simulink model "path_following_PID_v2"  (R2022a)
settings: Solver=VariableStepAuto  StartTime=0.0  StopTime=4000  RelTol=1e-3
model workspace (MAT data in the model file):
  index = 1
values from neighbouring files (symbols this model uses):
  ref = [x_ref, -y_ref]    [reference.m]
libraries: slpidlib x2
settings Model: Creator=andreagottardini  LastModifiedBy=andreagottardini
settings DataIOCC: ReturnWorkspaceOutputs=off

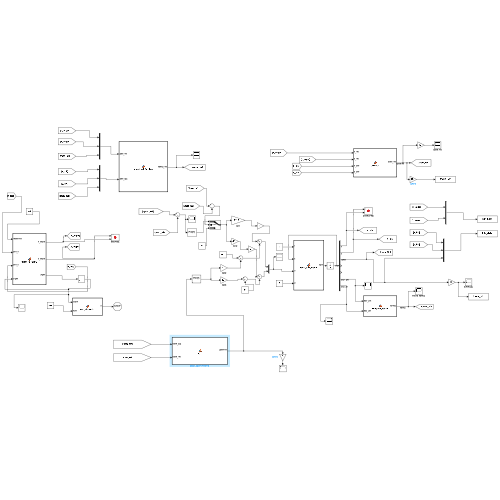
[thumbnail: Simulink's stored preview of the top-level diagram]
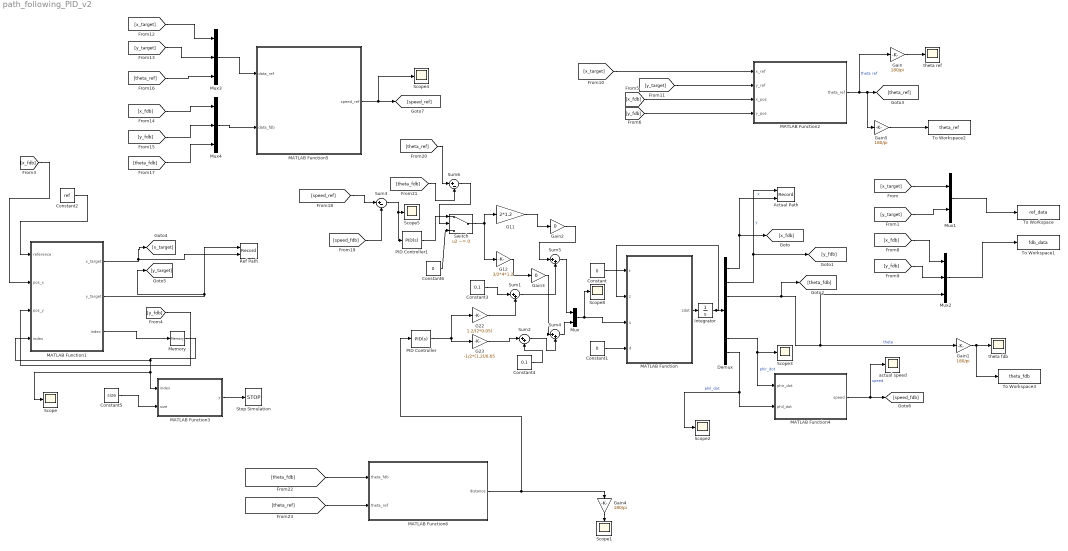
== system path_following_PID_v2 ==
  Actual Path : Record  FileSettingsInternal="{\"entries\":[{\"content\":{\"excelSettings\":{\"content\":{},\"type\":\"Streamout.ExcelSettings\"}},\"type\":\"Streamout.FileSettingStorage\",\"uuid\":\"b8018b94-6d69-4510-834d-5395391f9d9a\"}],\"packageUris\":[\"http://schema.mathworks.com/mf0/streamout_blocks/R2020a\"],\"version\":\"1.0\"}"  Layout=[1 1]  SignalsInternal="{\"entries\":[{\"content\":{\"signals\":[{\"content\":{\"blockPath\":[\"path_following_PID_v2/Actual Path\"],\"channel\":[],\"dimensions\":[1],\"domain\":\"path_following_PID_v2/Actual Path\",\"lineColor\":\"#22b573\",\"plots\":[],\"port\":1,\"sid\":[\"\"],\"signalID\":39276,\"signalName\":\"y\"},\"type\":\"RecordBlkView.Signal\",\"uuid\":\"de93c3ac-fa92-48e5-8615-195f95aa2750\"},{\"content\":{\"blockPath\":[\"path_following_PID_v2/Actual Path\"],\"channel\":[],\"dimensions\":[1],\"domain\":\"path_following_PID_v2/Actual Path\",\"lineColor\":\"#0072bd\",\"plots\":[],\"port\":2,\"sid\":[\"\"],\"signalID\":39280,\"signalName\":\"x\"},\"type\":\"RecordBlkView.Signal\",\"uuid\":\"afc86004-265b-4bb5-8c2d-c825a62d9dd9\"}]},\"type\":\"RecordBlkView.InputSignals\",\"uuid\":\"867639a0-b77e-437d-b3b9-b5e698d5be3f\"}],\"packageUris\":[\"http://schema.mathworks.com/mf0/streamout_blocks/R2020a\"],\"version\":\"1.0\"}"  VisualizationBindings="{\"xyplotplugin\":{\"info\":[{\"series\":[],\"subplotID\":1}]}}"  CompatibilityTag=XY
  Constant : Constant  Value=0
  Constant1 : Constant  Value=0
  Constant2 : Constant  Value=ref
  Constant3 : Constant  Value=0.1
  Constant4 : Constant  Value=0.1
  Constant5 : Constant  Value=size
  Constant6 : Constant  Value=0
  Demux : Demux  Outputs=7
  G11 : Gain  Gain=2*1.2
  G12 : Gain  Gain=3/2*4*1.2
  G22 : Gain  Gain=1.2/(2*0.05)
  G23 : Gain  Gain=-1/2*(1.2)/0.05
  Gain{,1,4..5} (4 alike) : Gain  Gain=180/pi
  Gain2 : Gain  Gain=0
  Gain3 : Gain  Gain=0
  Integrator : Integrator  InitialCondition=[0;0;0;0;0;0;0]
  MATLAB Function : MATLAB Function  TreatAsAtomicUnit=on
  MATLAB Function1 : MATLAB Function  TreatAsAtomicUnit=on
  MATLAB Function2 : MATLAB Function  TreatAsAtomicUnit=on
  MATLAB Function3 : MATLAB Function  TreatAsAtomicUnit=on
  MATLAB Function4 : MATLAB Function  TreatAsAtomicUnit=on
  MATLAB Function5 : MATLAB Function  TreatAsAtomicUnit=on
  MATLAB Function6 : MATLAB Function  TreatAsAtomicUnit=on
  Memory : Memory  InitialCondition=1
  Mux : Mux  Inputs=2
  Mux1 : Mux  Inputs=2
  Mux2 : Mux  Inputs=3
  Mux3 : Mux  Inputs=3
  Mux4 : Mux  Inputs=3
  PID Controller : slpidlib/PID Controller  Controller=PID  Form=Parallel  TimeDomain=Continuous-time  UseExternalTs=off  SampleTime=-1  IntegratorMethod=Forward Euler  FilterMethod=Forward Euler  ControllerParametersSource=internal  P=0.154648125989768  I=0.0265164152640643  UseKiTs=off  D=0.207345153563612  N=572.770791824146  UseFilter=on  TunerSelectOption=Frequency Response Based  InitialConditionSource=internal  InitialConditionForIntegrator=0  InitialConditionForFilter=0  DifferentiatorICPrevScaledInput=0  ExternalReset=none  TrackingMode=off  Kt=1  LimitOutput=off  SatLimitsSource=internal  UpperSaturationLimit=inf  LowerSaturationLimit=-inf  LinearizeAsGain=on  AntiWindupMode=none  Kb=1  POutMin=[]  POutMax=[]  IOutMin=[]  IOutMax=[]  DOutMin=[]  DOutMax=[]  NOutMin=[]  NOutMax=[]  SumOutMin=[]  SumOutMax=[]  SaturationOutMin=[]  SaturationOutMax=[]  PParamMin=[]  PParamMax=[]  IParamMin=[]  IParamMax=[]  DParamMin=[]  DParamMax=[]  NParamMin=[]  NParamMax=[]  KbParamMin=[]  KbParamMax=[]  KtParamMin=[]  KtParamMax=[]  KbOutMin=[]  KbOutMax=[]  KtOutMin=[]  KtOutMax=[]  IntegratorOutMin=[]  IntegratorOutMax=[]  FilterOutMin=[]  FilterOutMax=[]  SumI1OutMin=[]  SumI1OutMax=[]  SumI2OutMin=[]  SumI2OutMax=[]  SumI3OutMin=[]  SumI3OutMax=[]  SumI4OutMin=[]  SumI4OutMax=[]  SumDOutMin=[]  SumDOutMax=[]  DifferentiatorOutMin=[]  DifferentiatorOutMax=[]  FilterDiffOutCoefMin=[]  FilterDiffOutCoefMax=[]  ReciprocalOutMin=[]  ReciprocalOutMax=[]  SumDenOutMin=[]  SumDenOutMax=[]  SumNumOutMin=[]  SumNumOutMax=[]  DivideOutMin=[]  DivideOutMax=[]  UdiffTsProdOutMin=[]  UdiffTsProdOutMax=[]  NTsProdOutMin=[]  NTsProdOutMax=[]  UintegralTsProdOutMin=[]  UintegralTsProdOutMax=[]  UngainTsProdOutMin=[]  UngainTsProdOutMax=[]  IntegratorContinuousStateAttributes=''  IntegratorStateMustResolveToSignalObject=off  IntegratorRTWStateStorageClass=Auto  FilterContinuousStateAttributes=''  FilterStateMustResolveToSignalObject=off  FilterRTWStateStorageClass=Auto  ParallelPVariant=InternalParameters  IdealPVariant=Disabled  IVariant=InternalParameters  DVariant=InternalParameters  IntegratorVariant=Continuous  SatVariant=Disabled  AWVariant=Passthrough  PCopyVariant=Disabled  TRVariant=Disabled  FdbkBlocksVariant=Forward  IdealPFdbkVariant=Disabled  SatFdbkVariant=Disabled  DerivativeFilterVariant=ContFilter  NVariant=InternalParameters  NCopyVariant=Disabled  FilterICVariant=InternalICsFilter  IntegratorICVariant=InternalICs  ExternalResetVariant=Disabled  TRSumVariant=Passthrough  SumFdbkVariant=Disabled  SumVariant=Sum_PID  TsampFilterVariant=InternalTs  TsampNgainVariant=Passthrough  TsampIntegralVariant=Passthrough  ExternalSaturationOutDataTypeStr=Inherit: Same as second input  aMode=0
  PID Controller1 : slpidlib/PID Controller  Controller=PID  Form=Parallel  TimeDomain=Continuous-time  UseExternalTs=off  SampleTime=-1  IntegratorMethod=Forward Euler  FilterMethod=Forward Euler  ControllerParametersSource=internal  P=0.5  I=0.01  UseKiTs=off  D=0.5  N=100  UseFilter=on  TunerSelectOption=Frequency Response Based  InitialConditionSource=internal  InitialConditionForIntegrator=0  InitialConditionForFilter=0  DifferentiatorICPrevScaledInput=0  ExternalReset=none  TrackingMode=off  Kt=1  LimitOutput=off  SatLimitsSource=internal  UpperSaturationLimit=inf  LowerSaturationLimit=-inf  LinearizeAsGain=on  AntiWindupMode=none  Kb=1  POutMin=[]  POutMax=[]  IOutMin=[]  IOutMax=[]  DOutMin=[]  DOutMax=[]  NOutMin=[]  NOutMax=[]  SumOutMin=[]  SumOutMax=[]  SaturationOutMin=[]  SaturationOutMax=[]  PParamMin=[]  PParamMax=[]  IParamMin=[]  IParamMax=[]  DParamMin=[]  DParamMax=[]  NParamMin=[]  NParamMax=[]  KbParamMin=[]  KbParamMax=[]  KtParamMin=[]  KtParamMax=[]  KbOutMin=[]  KbOutMax=[]  KtOutMin=[]  KtOutMax=[]  IntegratorOutMin=[]  IntegratorOutMax=[]  FilterOutMin=[]  FilterOutMax=[]  SumI1OutMin=[]  SumI1OutMax=[]  SumI2OutMin=[]  SumI2OutMax=[]  SumI3OutMin=[]  SumI3OutMax=[]  SumI4OutMin=[]  SumI4OutMax=[]  SumDOutMin=[]  SumDOutMax=[]  DifferentiatorOutMin=[]  DifferentiatorOutMax=[]  FilterDiffOutCoefMin=[]  FilterDiffOutCoefMax=[]  ReciprocalOutMin=[]  ReciprocalOutMax=[]  SumDenOutMin=[]  SumDenOutMax=[]  SumNumOutMin=[]  SumNumOutMax=[]  DivideOutMin=[]  DivideOutMax=[]  UdiffTsProdOutMin=[]  UdiffTsProdOutMax=[]  NTsProdOutMin=[]  NTsProdOutMax=[]  UintegralTsProdOutMin=[]  UintegralTsProdOutMax=[]  UngainTsProdOutMin=[]  UngainTsProdOutMax=[]  IntegratorContinuousStateAttributes=''  IntegratorStateMustResolveToSignalObject=off  IntegratorRTWStateStorageClass=Auto  FilterContinuousStateAttributes=''  FilterStateMustResolveToSignalObject=off  FilterRTWStateStorageClass=Auto  ParallelPVariant=InternalParameters  IdealPVariant=Disabled  IVariant=InternalParameters  DVariant=InternalParameters  IntegratorVariant=Continuous  SatVariant=Disabled  AWVariant=Passthrough  PCopyVariant=Disabled  TRVariant=Disabled  FdbkBlocksVariant=Forward  IdealPFdbkVariant=Disabled  SatFdbkVariant=Disabled  DerivativeFilterVariant=ContFilter  NVariant=InternalParameters  NCopyVariant=Disabled  FilterICVariant=InternalICsFilter  IntegratorICVariant=InternalICs  ExternalResetVariant=Disabled  TRSumVariant=Passthrough  SumFdbkVariant=Disabled  SumVariant=Sum_PID  TsampFilterVariant=InternalTs  TsampNgainVariant=Passthrough  TsampIntegralVariant=Passthrough  ExternalSaturationOutDataTypeStr=Inherit: Same as second input  aMode=0
  Ref Path : Record  FileSettingsInternal="{\"entries\":[{\"content\":{\"excelSettings\":{\"content\":{},\"type\":\"Streamout.ExcelSettings\"}},\"type\":\"Streamout.FileSettingStorage\",\"uuid\":\"c3dc1af7-2476-41f5-b106-07b005e75dba\"}],\"packageUris\":[\"http://schema.mathworks.com/mf0/streamout_blocks/R2020a\"],\"version\":\"1.0\"}"  Layout=[1 1]  SignalsInternal="{\"entries\":[{\"content\":{\"signals\":[{\"content\":{\"blockPath\":[\"path_following_PID_v2/Ref Path\"],\"channel\":[],\"dimensions\":[1],\"domain\":\"path_following_PID_v2/Ref Path\",\"lineColor\":\"#d95319\",\"plots\":[],\"port\":1,\"sid\":[\"\"],\"signalID\":39284,\"signalName\":\"MATLAB Function1:2\"},\"type\":\"RecordBlkView.Signal\",\"uuid\":\"17033721-a681-4952-9c41-d7b7f67aaf11\"},{\"content\":{\"blockPath\":[\"path_following_PID_v2/Ref Path\"],\"channel\":[],\"dimensions\":[1],\"domain\":\"path_following_PID_v2/Ref Path\",\"lineColor\":\"#edb120\",\"plots\":[],\"port\":2,\"sid\":[\"\"],\"signalID\":39288,\"signalName\":\"MATLAB Function1:1\"},\"type\":\"RecordBlkView.Signal\",\"uuid\":\"4bb31dce-2a51-4ba4-bee2-83ac67841100\"}]},\"type\":\"RecordBlkView.InputSignals\",\"uuid\":\"db265190-be58-4162-951c-6f002e6dceb6\"}],\"packageUris\":[\"http://schema.mathworks.com/mf0/streamout_blocks/R2020a\"],\"version\":\"1.0\"}"  VisualizationBindings="{\"xyplotplugin\":{\"info\":[{\"series\":[],\"subplotID\":1}]}}"  CompatibilityTag=XY
  Scope{,1..5,8} (7 alike) : Scope
  Stop Simulation : Stop
  Sum{1..2,4..5} (4 alike) : Sum  Inputs=|++
  Sum3 : Sum  Inputs=|+-
  Sum6 : Sum  Inputs=|+-
  Switch : Switch  Criteria=u2 ~= 0  SaturateOnIntegerOverflow=off  InputSameDT=off
  To Workspace : ToWorkspace  VariableName=ref_data  SampleTime=-1
      settings: Save2DSignal=2-D array (concatenate along first dimension)
  To Workspace1 : ToWorkspace  VariableName=fdb_data  SampleTime=-1
      settings: Save2DSignal=2-D array (concatenate along first dimension)
  To Workspace2 : ToWorkspace  VariableName=theta_ref  SaveFormat=Timeseries  SampleTime=-1
  To Workspace3 : ToWorkspace  VariableName=theta_fdb  SaveFormat=Timeseries  SampleTime=-1
  actual speed : Scope
  theta fdb : Scope
  theta ref : Scope
  wires:
  Constant/1 -> MATLAB Function/1(t)
  Constant1/1 -> MATLAB Function/4(d)
  Integrator/1 -> MATLAB Function/2(z), Demux/1
  MATLAB Function/1(zdot) -> Integrator/1
  PID Controller/1 -> G22/1, G23/1
  Demux/1 -> Actual Path/2, [x_fdb]  "x"
  Demux/2 -> Actual Path/1, [y_fdb]  "y"
  Demux/3 -> Mux2/3, Gain1/1, [theta_fdb]  "theta"
  MATLAB Function1/1(x_target) -> [x_target], Ref Path/2
  Constant2/1 -> MATLAB Function1/1(reference)
  [x_fdb] -> MATLAB Function1/2(pos_x)
  [y_fdb] -> MATLAB Function1/3(pos_y)
  [x_fdb] -> MATLAB Function2/3(x_pos)
  [y_fdb] -> MATLAB Function2/4(y_pos)
  MATLAB Function2/1(theta_ref) -> Gain/1, Gain5/1, [theta_ref]  "theta ref"
  MATLAB Function1/2(y_target) -> Ref Path/1, [y_target]
  [x_target] -> MATLAB Function2/1(x_ref)
  [y_target] -> MATLAB Function2/2(y_ref)
  Memory/1 -> Scope/1, MATLAB Function3/1(index), MATLAB Function1/4("index ")
  MATLAB Function1/3(index) -> Memory/1
  Constant5/1 -> MATLAB Function3/2(size)
  MATLAB Function3/1(y) -> Stop Simulation/1
  Sum1/1 -> Sum5/2
  Sum2/1 -> Sum4/2
  G22/1 -> Sum1/2
  G23/1 -> Sum2/1
  Constant3/1 -> Sum1/1
  Constant4/1 -> Sum2/2
  [y_fdb] -> Mux2/2
  [x_fdb] -> Mux2/1
  [y_target] -> Mux1/2
  [x_target] -> Mux1/1
  Mux1/1 -> To Workspace/1
  Mux2/1 -> To Workspace1/1
  Demux/6 -> MATLAB Function4/1(phir_dot), Scope3/1  "phir_dot"
  Demux/7 -> Scope2/1, MATLAB Function4/2(phil_dot)  "phil_dot"
  MATLAB Function4/1(speed) -> actual speed/1, [speed_fdb]  "speed"
  [theta_ref] -> Mux3/3
  [x_target] -> Mux3/1
  [y_target] -> Mux3/2
  Mux3/1 -> MATLAB Function5/1(data_ref)
  [x_fdb] -> Mux4/1
  [y_fdb] -> Mux4/2
  [theta_fdb] -> Mux4/3
  Mux4/1 -> MATLAB Function5/2(data_fdb)
  MATLAB Function5/1(speed_ref) -> Scope4/1, [speed_ref]
  [speed_ref] -> Sum3/1
  [speed_fdb] -> Sum3/2
  Sum3/1 -> Scope5/1, PID Controller1/1
  Mux/1 -> Scope8/1, MATLAB Function/3(u)
  Sum4/1 -> Mux/2
  Sum5/1 -> Mux/1
  Switch/1 -> G11/1, G12/1
  PID Controller1/1 -> Switch/1
  Constant6/1 -> Switch/3
  Sum6/1 -> Switch/2
  [theta_ref] -> Sum6/1
  [theta_fdb] -> Sum6/2
  Gain/1 -> theta ref/1
  Gain1/1 -> To Workspace3/1, theta fdb/1
  [theta_fdb] -> MATLAB Function6/1(theta_fdb)
  [theta_ref] -> MATLAB Function6/2(theta_ref)
  MATLAB Function6/1(distance) -> PID Controller/1, Gain4/1
  G11/1 -> Gain2/1
  Gain2/1 -> Sum5/1
  G12/1 -> Gain3/1
  Gain3/1 -> Sum4/1
  Gain4/1 -> Scope1/1
  Gain5/1 -> To Workspace2/1

== matlab function path_following_PID_v2/MATLAB Function1 ==
  data: reference input; x_target output; pos_x input; pos_y input; y_target output; index input; index output
function [x_target, y_target, index] = target_to_follow(reference, pos_x, pos_y,index)

current_target_x = reference(index,1);
current_target_y = reference(index,2);

distance = sqrt((current_target_x - pos_x)^2+(current_target_y - pos_y)^2);

if distance <= 0.5
    index= index + 1;
else
    index = index;
end


x_target = reference(index,1);
y_target = reference(index,2);


end

== matlab function path_following_PID_v2/MATLAB Function ==
  data: t input; z input; u input; zdot output; d input
function zdot=robot_dyn_model(t,z,u,d)

%% Read parameters, states and inputs

% Parameters
% Ic      =       th(1,1);     %
% Iw      =       th(2,1);     % 
% d       =       th(3,1);     % 
% mw      =       th(4,1);     % 
% mc      =       th(5,1);     % 
% Im      =       th(6,1);     % 
% R       =       th(7,1);     % 
% L       =       th(8,1);     % 

 Ic      =       1;     %
 Iw      =       0.1;     % 
 d       =       0.05;     % 
 mw      =       0.1;     % 
 mc      =       1;     % 
 Im      =       0.1;     % 
 R       =       0.025;     % 
 L       =       0.05;

mT = mc+2*mw;
I = Ic+mc*d^2+2*mw*L^2+2*Im;


% States
xa                  =       z(1,1);    % inertial X position (m)
ya                  =       z(2,1);    % inertial Y position (m)
theta               =       z(3,1);    % body orientation - yaw angle(rad)
phir                =       z(4,1);    % angular displacement right wheel (rad)
phil                =       z(5,1);    % angular displacement left wheel (rad)
phir_dot            =       z(6,1);    % angular velocity right wheel (rad/s)    
phil_dot            =       z(7,1);    % angular velocity left wheel (rad/s)



% Additional paramaeters
cth = cos(theta);
sth = sin(theta);

lam = [-sth     cth     0;
        cth     sth     L;
        cth     sth     -L];

b = inv(lam)*[0; R*phir_dot; R*phil_dot];

xa_dot      =    b(1,1);
ya_dot      =    b(2,1);
theta_dot   =    b(3,1);




% Inputs
taur      =       u(1,1);     % driving/braking torque right wheel (N*m)
taul      =       u(2,1);     % driving/braking torque left wheel (N*m)


%% Matrices


S = [R/(2*L)*(L*cth-d*sth) R/(2*L)*(L*cth+d*sth);
     R/(2*L)*(L*sth+d*cth) R/(2*L)*(L*sth-d*cth);
     R/(2*L)               -R/(2*L)             ;
     1                      0                   ;
     0                      1];


M_bar = [Iw+R^2/(4*L^2)*(mT*L^2+I)          R^2/(4*L^2)*(mT*L^2-I); 
        R^2/(4*L^2)*(mT*L^2-I)              Iw+R^2/(4*L^2)*(mT*L^2+I)];

V_bar = [0                              R^2/(2*L)*mc*d*theta_dot;
        -R^2/(2*L)*mc*d*theta_dot               0];



% Model equations

zdot = zeros(7,1);

zdot = [S*z(6:7,1); zeros(2,1)] + [zeros(5,2); eye(2)]*inv(M_bar)*(u-V_bar*z(6:7,1));

== matlab function path_following_PID_v2/MATLAB Function2 ==
  data: x_ref input; theta_ref output; y_ref input; x_pos input; y_pos input
function theta_ref = direction (x_ref, y_ref, x_pos, y_pos)

if (x_pos >= x_ref && abs(y_pos-y_ref)<=10^-3)
    theta_ref = pi;
elseif (abs(x_pos-x_ref)<=10^-3 && y_pos <= y_ref )
    theta_ref = pi/2;
elseif (x_pos < x_ref && abs(y_pos-y_ref)<=10^-3)
    theta_ref = 0;
elseif (abs(x_pos-x_ref)<=10^-3 && y_pos > y_ref )
    theta_ref = 3*pi/2;
elseif (x_pos<x_ref && y_pos<y_ref)
    theta_ref = atan((y_ref-y_pos)/(x_ref-x_pos));
elseif (x_pos>x_ref && y_pos<y_ref)
    theta_ref = pi-atan((y_ref-y_pos)/(x_pos-x_ref));
elseif (x_pos>x_ref && y_pos>y_ref)
    theta_ref = pi+atan((y_pos-y_ref)/(x_pos-x_ref));
else %(x_pos<x_ref && y_pos>y_ref)
    theta_ref = 2*pi-atan((y_pos-y_ref)/(x_ref-x_pos));
end





% if (theta_fdb<0)
%     theta_fdb=theta_fdb+2*pi;
% end
% 
% distance_clockwise = 2*pi-theta_ref1+theta_fdb;
% distance_anticlockwise = theta_ref1-theta_fdb;
% 
% 
% if (distance_clockwise<=distance_anticlockwise) %girare clockwise
%     theta_ref = theta_ref1-2*pi;
% else %girare anticlockwise
%     theta_ref = theta_ref1;
% end
% 
% 
% end

== matlab function path_following_PID_v2/MATLAB Function3 ==
  data: index input; y output; size input
function y = stop_simulation(index, size)

if (index == size)
    y = 1;
else 
    y=0;

end

== matlab function path_following_PID_v2/MATLAB Function4 ==
  data: phir_dot input; speed output; phil_dot input
function speed = compute_speed(phir_dot, phil_dot)

speed = ((phir_dot*0.025)+(phil_dot*0.025))/2;

== matlab function path_following_PID_v2/MATLAB Function5 ==
  data: data_ref input; data_fdb input; speed_ref output
function speed_ref = speed_ref_function(data_ref, data_fdb)

x_ref = data_ref(1);
y_ref = data_ref(2);
theta_ref = data_ref(3);

x_fdb = data_fdb(1);
y_fdb = data_fdb(2);
theta_fdb = data_fdb(3);


distance = sqrt((x_ref-x_fdb)^2+(y_ref-y_fdb)^2);


% if (abs(theta_ref-theta_fdb)<=pi/30)
%     c=5;
% else 
%     c=5/abs(theta_ref-theta_fdb);
% end

speed = 0.4*distance;

if speed >= 1.6
    speed_ref = 1.6;
else 
    speed_ref = speed;
end

== matlab function path_following_PID_v2/MATLAB Function6 ==
  data: theta_fdb input; theta_ref input; distance output
function distance = fcn(theta_fdb,theta_ref)

% 
% if (theta_fdb<0)
%     theta_fdb=theta_fdb+2*pi;
% end
% 
% distance_clockwise = 2*pi-theta_ref+theta_fdb;
% distance_anticlockwise = theta_ref-theta_fdb;
% 
% if (distance_clockwise<=distance_anticlockwise)
%     y = -1;
%     distance = y*distance_clockwise;
% else
%     y = 1;
%     distance = y*distance_anticlockwise;
% end



distance = rem((theta_ref - theta_fdb),2*pi);
if (distance < -pi)
    distance = (distance + 2*pi);
elseif (distance > pi)
    distance = (distance - 2*pi);

end
